simulink model "model_mass_spring_damper_estimate"  (R2021a)
settings: Solver=VariableStepAuto  StartTime=0.0  StopTime=5  MaxStep=0.025  RelTol=1e-3  AbsTol=1e-3  EnableMultiTasking=on
PreLoadFcn:
  | init_mass_spring_damper_estimate;
values from neighbouring files (symbols this model uses):
  estimates_b1 = 1    [init_mass_spring_damper_estimate.m]
  estimates_b2 = 1    [init_mass_spring_damper_estimate.m]
libraries: fl_lib x9, nesl_utility x3
Description:
  | Mass-Spring-Damper in Simulink(R) and Simscape(TM)
settings Model: OrderedModelArguments=off  Creator=The MathWorks, Inc.  LastModifiedBy=ytang
settings SolverCC: AutoScaleAbsTol=off  AlgebraicLoopSolver=TrustRegion
settings DataIOCC: LimitDataPoints=on  SaveFormat=Array  ReturnWorkspaceOutputs=off  SignalLoggingName=logsout_ssc_mass_spring_damper_sl
settings OptimizationCC: LifeSpan=inf
settings DebuggingCC: SolverPrmCheckMsg=warning  AllowSymbolicDim=off  PregeneratedLibrarySubsystemCodeDiagnostic=none  SFUnexpectedBacktrackingDiag=warning  SFNoUnconditionalDefaultTransitionDiag=warning  SFExecutionAtInitializationDiag=none  SFMachineParentedDataDiag=warning  ArithmeticOperatorsInVariantConditions=warning
settings HardwareCC: ProdBitPerPointer=32  ProdBitPerSizeT=32  ProdBitPerPtrDiffT=32  ProdLargestAtomicFloat=None  ProdIntDivRoundTo=Undefined  ProdEndianess=Unspecified  ProdWordSize=32  ProdHWDeviceType=32-bit Generic
settings ModelReferenceCC: PropagateSignalLabelsOutOfModel=off
settings SFSimCC: SimUseLocalCustomCode=off  CustomCodeUndefinedFunction=UseInterfaceOnly
settings RTWCC: RTWUseLocalCustomCode=off
settings CodeAppCC: StateflowObjectComments=on
settings GRTTargetCC: TargetLangStandard=C89/C90 (ANSI)
settings ConfigComp: CovMetricSettings=dw  CovSaveCumulativeToWorkspaceVar=on  CovSaveSingleToWorkspaceVar=on  CovExternalEMLEnable=off  CovSFcnEnable=off
settings SimscapeCC: SimscapeLogType=all  SimscapeLogLimitData=off  SimscapeLogDataHistory=10000

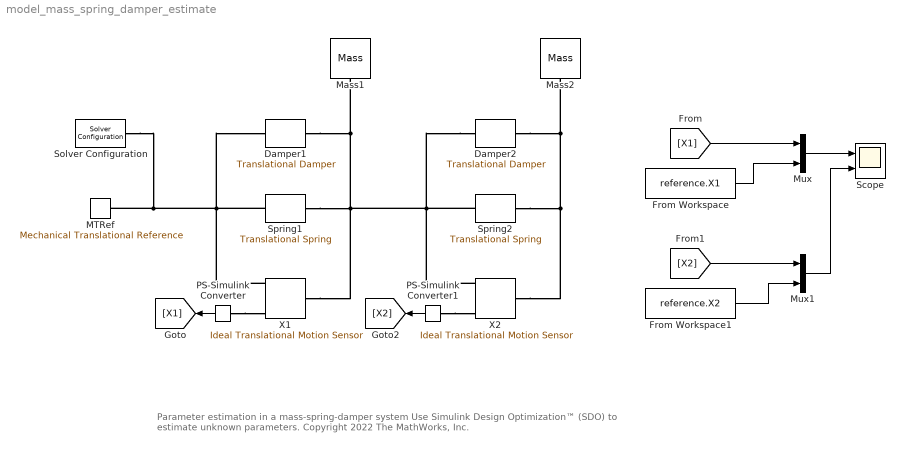
== system model_mass_spring_damper_estimate ==
  note: Parameter estimation in a mass-spring-damper system
      |
      | Use Simulink Design Optimization™ (SDO) to estimate unknown parameters.
      |
      | Copyright 2022 The MathWorks, Inc.
  Damper1 : fl_lib/Mechanical/Translational Elements/Translational Damper  D=estimates_b1 N/(m/s)  v_specify=off  v_priority=High  v=0 m/s  v_nominal_specify=off  v_nominal_unit=m/s  v_nominal_value=1  f_specify=off  f_priority=High  f=0 N  f_nominal_specify=off  f_nominal_unit=N  f_nominal_value=1
  Damper2 : fl_lib/Mechanical/Translational Elements/Translational Damper  D=estimates_b2 N/(m/s)  v_specify=off  v_priority=High  v=0 m/s  v_nominal_specify=off  v_nominal_unit=m/s  v_nominal_value=1  f_specify=off  f_priority=High  f=0 N  f_nominal_specify=off  f_nominal_unit=N  f_nominal_value=1
  From Workspace : FromWorkspace  VariableName=reference.X1
  From Workspace1 : FromWorkspace  VariableName=reference.X2
  MTRef : fl_lib/Mechanical/Translational Elements/Mechanical Translational Reference
  Mass1 : fl_lib/Mechanical/Translational Elements/Mass  mass=estimates_m1 kg  num_ports=foundation.enum.numPorts2.one  v_specify=off  v_priority=High  v=0 m/s  v_nominal_specify=off  v_nominal_unit=m/s  v_nominal_value=1  f_specify=off  f_priority=High  f=0 N  f_nominal_specify=off  f_nominal_unit=N  f_nominal_value=1
  Mass2 : fl_lib/Mechanical/Translational Elements/Mass  mass=estimates_m2 kg  num_ports=foundation.enum.numPorts2.one  v_specify=off  v_priority=High  v=0 m/s  v_nominal_specify=off  v_nominal_unit=m/s  v_nominal_value=1  f_specify=off  f_priority=High  f=0 N  f_nominal_specify=off  f_nominal_unit=N  f_nominal_value=1
  Mux : Mux  Inputs=2
  Mux1 : Mux  Inputs=2
  PS-Simulink Converter : nesl_utility/PS-Simulink Converter  PhysicalDomain=network_engine_domain  SubClassName=ps_output  LeftPortType=input  RightPortType=output  PseudoPeriodic=off  Frequencies=[]  Unit=m  AffineConversion=off
      settings: SourceProductBaseCode=PW,SS
  PS-Simulink Converter1 : nesl_utility/PS-Simulink Converter  PhysicalDomain=network_engine_domain  SubClassName=ps_output  LeftPortType=input  RightPortType=output  PseudoPeriodic=off  Frequencies=[]  Unit=m  AffineConversion=off
      settings: SourceProductBaseCode=PW,SS
  Scope : Scope  NumInputPorts=2
  Solver Configuration : nesl_utility/Solver Configuration  PhysicalDomain=network_engine_domain  SubClassName=solver  LeftPortType=input  RightPortType=generic  Tones=[]  Harmonics=[]  SimulateNoise=off  Profile=off  UseLocalSampling=off  EnableSwitchedLinearOptims=on  FrequencyDomain=off  UseCCode=off  RelTol=0.001  AbsTol=1e-06  MinStep=1e-09  ToWorkspace=off  RevertToSquareIcSolve=off  NumHomotopyIterations=100  PhasorMode=off  PhasorModeNumHarmonics=1  DoDC=off  ResidualTolerance=1e-9  UseLocalSolver=off  LocalSolverChoice=NE_BACKWARD_EULER_ADVANCER  LocalSolverSampleTime=.001  DoFixedCost=off  MaxNonlinIter=12  MaxModeIter=2  ComputeImpulses=off  ImpulseIterations=2  LinearAlgebra=auto  EquationFormulation=NE_TIME_EF  DelaysMemoryBudget=1024  AutomaticFiltering=on  FilteringTimeConstant=0.001  PartitionStorageMethod=AS_NEEDED  PartitionMemoryBudget=1024  PartitionMethod=FAST
      settings: SourceProductBaseCode=PW,SS
  Spring1 : fl_lib/Mechanical/Translational Elements/Translational Spring  spr_rate=estimates_k1 N/m  v_specify=off  v_priority=High  v=0 m/s  v_nominal_specify=off  v_nominal_unit=m/s  v_nominal_value=1  f_specify=off  f_priority=High  f=0 N  f_nominal_specify=off  f_nominal_unit=N  f_nominal_value=1  x_specify=on  x_priority=High  x=estimates_x1 m  x_nominal_specify=off  x_nominal_unit=m  x_nominal_value=1
  Spring2 : fl_lib/Mechanical/Translational Elements/Translational Spring  spr_rate=estimates_k2 N/m  v_specify=off  v_priority=High  v=0 m/s  v_nominal_specify=off  v_nominal_unit=m/s  v_nominal_value=1  f_specify=off  f_priority=High  f=0 N  f_nominal_specify=off  f_nominal_unit=N  f_nominal_value=1  x_specify=on  x_priority=High  x=estimates_x2 m  x_nominal_specify=off  x_nominal_unit=m  x_nominal_value=1
  X1 : fl_lib/Mechanical/Mechanical Sensors/Ideal Translational Motion Sensor  offset=estimates_x1 m
  X2 : fl_lib/Mechanical/Mechanical Sensors/Ideal Translational Motion Sensor  offset=estimates_x2 m
  wires:
  From Workspace/1 -> Mux/2
  Mux/1 -> Scope/1
  PS-Simulink Converter/1 -> [X1]
  [X1] -> Mux/1
  PS-Simulink Converter1/1 -> [X2]
  [X2] -> Mux1/1
  From Workspace1/1 -> Mux1/2
  Mux1/1 -> Scope/2
  connections:
  X1/RConn1 -- Spring1/RConn1 -- Damper1/RConn1 -- Solver Configuration/RConn1 -- MTRef/LConn1
  PS-Simulink Converter/LConn1 -- X1/RConn3
  Damper2/RConn1 -- Spring2/RConn1 -- X2/RConn1 -- Spring1/LConn1 -- Damper1/LConn1 -- Mass1/LConn1 -- X1/LConn1
  X2/LConn1 -- Spring2/LConn1 -- Mass2/LConn1 -- Damper2/LConn1
  PS-Simulink Converter1/LConn1 -- X2/RConn3
